simulink model "Modele_Projet_H2026_Gabarit"  (R2021a)
settings: Solver=FixedStepAuto  StartTime=0.0  StopTime=60  FixedStep=10e-6  RelTol=1e-3
InitFcn:
  | clear all
  | close all
  | 
  | % Chariot
  | 
  | M = 2.5 % [kg]
  | 
  | % Reducteur  / roue
  | 
  | G1 = 20        %  Rapport rédcuteur
  | r1  = 0.125     %  Rayon roue [m]
  | 
  | %Moteur 80ZYTC102-1 Brush DC Motor
  | 
  | uB = 24 % V
  | 
  | km = 0.0742   % Nm/A
  | 
  | kv =  0.0742 % V / (rad/s)
  | 
  | Lm = 1.577e-3 % H
  | 
  | Rm = 1.3    % Ohm
  | 
  | Jr = 1.5580e-04    % kg-m2
  | 
  | Jch =  M*r1^2/G1^2
  | 
  | Jm = Jr + Jch
  | 
  | Bm = 0.0015 % Nm.s
  | 
  | 
  | 
  | Cf = 300e-6  % F
  | 
  | Lf = 50e-6 %  H
  | 
  | Rf = 100000 % Ohm
  | 
  | 
  | % Couplage
  | k = 50   % Constante d'élasticité  [N/m]
  | 
  | 
  | 
  | % Parametre perso ajouté pour le test
  | 
  | 
  | uB = 24;            % [V]       Tension nominale de la batterie
  | 
  | 
  | %% -------------------------------------------------------------------------
  | %  2. MOTEUR À COURANT CONTINU  (80ZYTC102-1 Brush DC Motor)
  | %     Identique pour les deux chariots
  | %% -------------------------------------------------------------------------
  | Lm = 1.577e-3;      % [H]       Inductance de l'induit
  | Rm = 1.3;           % [Ohm]     Résistance de l'induit
  | km = 0.0742;        % [Nm/A]    Constante de couple
  | kv = 0.0742;        % [V.s/rad] Constante de tension (FEM)
  | Jr = 1.558e-4;      % [kg.m²]   Inertie du rotor (avec charge)
  | Bm = 1.5e-3;        % [Nm.s]    Coefficient de friction visqueuse
  | 
  | 
  | %% -------------------------------------------------------------------------
  | %  3. CHARIOT
  | %% -------------------------------------------------------------------------
  | M  = 2.5;           % [kg]      Masse d'un chariot
  | G  = 20;            % [-]       Rapport du réducteur de vitesse
  | r  = 0.125;         % [m]       Rayon des roues
  | 
  | 
  | %% -------------------------------------------------------------------------
  | %  4. FILTRE DU CONVERTISSEUR DE PUISSANCE
  | %% -------------------------------------------------------------------------
  | Cf = 300e-6;        % [F]       Condensateur du filtre
  | Lf = 50e-6;         % [H]       Inductance du filtre
  | Rf = 100e3;         % [Ohm]     Résistance du filtre
  | 
  | 
  | %% -------------------------------------------------------------------------
  | %  5. BANDE ÉLASTIQUE
  | %% -------------------------------------------------------------------------
  | k_elas = 50;        % [N/m]     Constante d'élasticité de la bande
  | L_band = 1;         % [m]       Longueur de la bande élastique
  | 
  | 
  | %% -------------------------------------------------------------------------
  | %  6. PARAMÈTRES CALCULÉS
  | %% -------------------------------------------------------------------------
  | 
  | 
  | % --- Inertie équivalente vue par le moteur (Éq. 4) ---
  | rG   = r / G;                           % [m/rad]   Gain cinématique = 0.00625
  | Jm   = Jr + M * rG^2;                   % [kg.m²]   = 2.535e-4
  | 
  | 
  | % --- Constantes de temps du moteur ---
  | tau_e = Lm / Rm;                        % [s]       Cste de temps électrique = 1.213e-3 s
  | tau_m = Jm / Bm;                        % [s]       Cste de temps mécanique  = 0.1690  s
  | 
  | 
  | % --- Produit des constantes moteur (FEM contre-réaction) ---
  | km_kv = km * kv;                        % [V.Nm/A²] = 5.506e-3
  | 
  | 
  | % --- Paramètres du modèle simplifié (tau_e négligé) ---
  | Bm_star  = Bm + km*kv/Rm;              % [Nm.s]    Friction équivalente = 5.737e-3
  | tau_m_st = Jm / Bm_star;               % [s]       Cste de temps simplifiée = 0.04418 s
  | Kv       = uB*km / (Rm * Bm_star);     % [rad/s]   Gain BO vitesse simplifié = 238.8
  | Kp       = Kv * rG;                     % [m/s]     Gain BO position simplifiée = 1.493
  | 
  | 
  | % --- Gain du convertisseur (simplifié) ---
  | K_conv = uB;                            % [V]       = 24  (gain pur)
  | 
  | 
  | % --- Gain cinématique couplage ---
  | rG_sq  = rG^2;
undefined symbols (not defined in the file or in its folder): sigbuilder_block
settings Model: Creator=cardenas  LastModifiedBy=arman

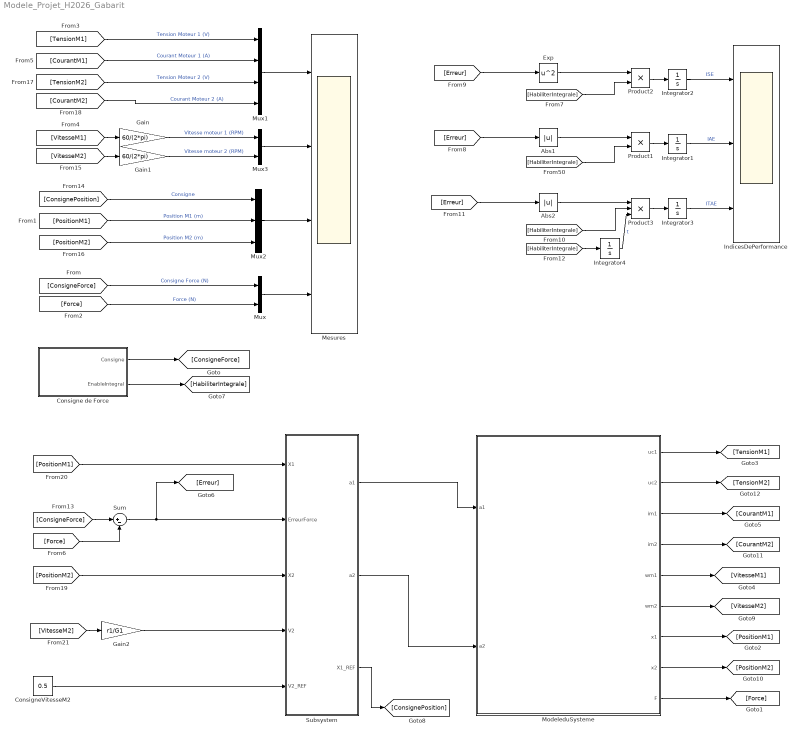
== system Modele_Projet_H2026_Gabarit ==
  Abs1 : Abs
  Abs2 : Abs
  Consigne de Force : Subsystem
  ConsigneVitesseM2 : Constant  Value=0.5
  Exp : Math  Operator=square  SaturateOnIntegerOverflow=on
  Gain : Gain  Gain=60/(2*pi)
  Gain1 : Gain  Gain=60/(2*pi)
  Gain2 : Gain  Gain=r1/G1
  IndicesDePerformance : Scope  NumInputPorts=3
  Integrator{1..4} (4 alike) : Integrator
  Mesures : Scope  NumInputPorts=4
  ModeleduSysteme : Subsystem
  Mux : Mux  Inputs=2
  Mux1 : Mux
  Mux2 : Mux  Inputs=3
  Mux3 : Mux  Inputs=2
  Product1 : Product
  Product2 : Product
  Product3 : Product  Inputs=3
  Subsystem : Subsystem
  Sum : Sum  Inputs=|+-
  wires:
  Mux/1 -> Mesures/4
  [ConsigneForce] -> Mux/1  "Consigne Force (N)"
  [PositionM1] -> Mux2/2  "Position M1 (m)"
  [Force] -> Mux/2  "Force (N)"
  [TensionM1] -> Mux1/1  "Tension Moteur 1 (V)"
  [VitesseM1] -> Gain/1
  Sum/1 -> [Erreur], Subsystem/2(ErreurForce)
  ModeleduSysteme/9(F) -> [Force]
  ModeleduSysteme/1(uc1) -> [TensionM1]
  ModeleduSysteme/7(x1) -> [PositionM1]
  ModeleduSysteme/3(im1) -> [CourantM1]
  [CourantM1] -> Mux1/2  "Courant Moteur 1 (A)"
  Mux1/1 -> Mesures/1
  ModeleduSysteme/5(wm1) -> [VitesseM1]
  [Force] -> Sum/2
  Gain/1 -> Mux3/1  "Vitesse moteur 1 (RPM)"
  [Erreur] -> Abs1/1
  [HabiliterIntegrale] -> Product1/2
  Abs1/1 -> Product1/1
  Product1/1 -> Integrator1/1
  Integrator1/1 -> IndicesDePerformance/2  "IAE"
  Product2/1 -> Integrator2/1
  Exp/1 -> Product2/1
  [HabiliterIntegrale] -> Product2/2
  Integrator2/1 -> IndicesDePerformance/1  "ISE"
  [Erreur] -> Exp/1
  Integrator3/1 -> IndicesDePerformance/3  "ITAE"
  Product3/1 -> Integrator3/1
  Abs2/1 -> Product3/1
  [HabiliterIntegrale] -> Product3/2
  [Erreur] -> Abs2/1
  Consigne de Force/2(EnableIntegral) -> [HabiliterIntegrale]
  [HabiliterIntegrale] -> Integrator4/1
  Integrator4/1 -> Product3/3  "t"
  [ConsigneForce] -> Sum/1
  [ConsignePosition] -> Mux2/1  "Consigne"
  Mux2/1 -> Mesures/3
  ModeleduSysteme/6(wm2) -> [VitesseM2]
  Mux3/1 -> Mesures/2
  Gain1/1 -> Mux3/2  "Vitesse moteur 2 (RPM)"
  [VitesseM2] -> Gain1/1
  ModeleduSysteme/8(x2) -> [PositionM2]
  [PositionM2] -> Mux2/3  "Position M2 (m)"
  ModeleduSysteme/4(im2) -> [CourantM2]
  ModeleduSysteme/2(uc2) -> [TensionM2]
  [TensionM2] -> Mux1/3  "Tension Moteur 2 (V)"
  [CourantM2] -> Mux1/4  "Courant Moteur 2 (A)"
  Consigne de Force/1(Consigne) -> [ConsigneForce]
  [VitesseM2] -> Gain2/1
  [PositionM1] -> Subsystem/1(X1)
  [PositionM2] -> Subsystem/3(X2)
  Gain2/1 -> Subsystem/4(V2)
  ConsigneVitesseM2/1 -> Subsystem/5(V2_REF)
  Subsystem/1(a1) -> ModeleduSysteme/1(a1)
  Subsystem/2(a2) -> ModeleduSysteme/2(a2)
  Subsystem/3(X1_REF) -> [ConsignePosition]

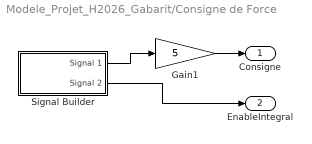
== system Modele_Projet_H2026_Gabarit/Consigne de Force ==
  Gain1 : Gain  Gain=5
  Signal Builder : Subsystem  Tag=STV Subsys  LoadFcn=sigbuilder_block('load');  StartFcn=sigbuilder_block('start');  StopFcn=sigbuilder_block('stop');  ClipboardFcn=sigbuilder_block('clipboard');  mask(Sigbuilder block){tuvar=[0:10]}
      mask help: Simulink:masks:SigbuilderBlock_MD
      mask init:
      | if ~strcmp(get_param(bdroot(gcbh),'SimulationStatus'),'stopped') tuvar = sigbuilder_block('maskInit'); end
      settings: CopyFcn=sigbuilder_block('copy');  DeleteFcn=sigbuilder_block('delete');  ModelCloseFcn=sigbuilder_block('modelClose');  PreSaveFcn=sigbuilder_block('preSave');  PauseFcn=sigbuilder_block('pause');  ContinueFcn=sigbuilder_block('continue');  NameChangeFcn=sigbuilder_block('namechange');  OpenFcn=sigbuilder_block('open',[138 164.25 838.5 442.5 ]);  CloseFcn=sigbuilder_block('close');
      mask Display: plot(0, 0, 100, 100,[2, 2, 32, 32, 2], [68, 8, 8, 68, 68],[32, 2], [38, 38], [32, 19, 2],[53, 60, 44], [32, 17, 17, 2],[16, 16, 31, 31]);txt = getActiveGroup(gcbh);text(2, 100, txt,'verticalAlignment', 'top');
  Consigne : Outport
  EnableIntegral : Outport  Port=2
  wires:
  Signal Builder/1(Signal 1) -> Gain1/1
  Gain1/1 -> Consigne/1
  Signal Builder/2(Signal 2) -> EnableIntegral/1

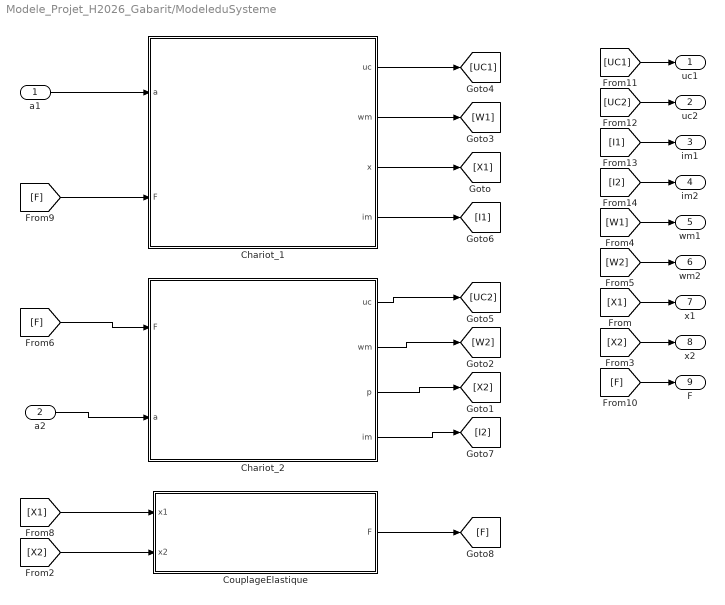
== system Modele_Projet_H2026_Gabarit/ModeleduSysteme ==
  a1 : Inport
  a2 : Inport  Port=2
  Chariot_1 : Subsystem
  Chariot_2 : Subsystem
  CouplageElastique : Subsystem
  uc1 : Outport
  uc2 : Outport  Port=2
  im1 : Outport  Port=3
  im2 : Outport  Port=4
  wm1 : Outport  Port=5
  wm2 : Outport  Port=6
  x1 : Outport  Port=7
  x2 : Outport  Port=8
  F : Outport  Port=9
  wires:
  CouplageElastique/1(F) -> [F]
  [X1] -> x1/1
  [X2] -> CouplageElastique/2(x2)
  [X2] -> x2/1
  [W1] -> wm1/1
  [W2] -> wm2/1
  Chariot_2/1(uc) -> [UC2]
  Chariot_2/2(wm) -> [W2]
  Chariot_2/3(p) -> [X2]
  Chariot_2/4(im) -> [I2]
  [F] -> Chariot_2/1(F)
  a2/1 -> Chariot_2/2(a)
  [X1] -> CouplageElastique/1(x1)
  [F] -> Chariot_1/2(F)
  Chariot_1/1(uc) -> [UC1]
  Chariot_1/2(wm) -> [W1]
  Chariot_1/3(x) -> [X1]
  Chariot_1/4(im) -> [I1]
  a1/1 -> Chariot_1/1(a)
  [F] -> F/1
  [UC1] -> uc1/1
  [UC2] -> uc2/1
  [I1] -> im1/1
  [I2] -> im2/1

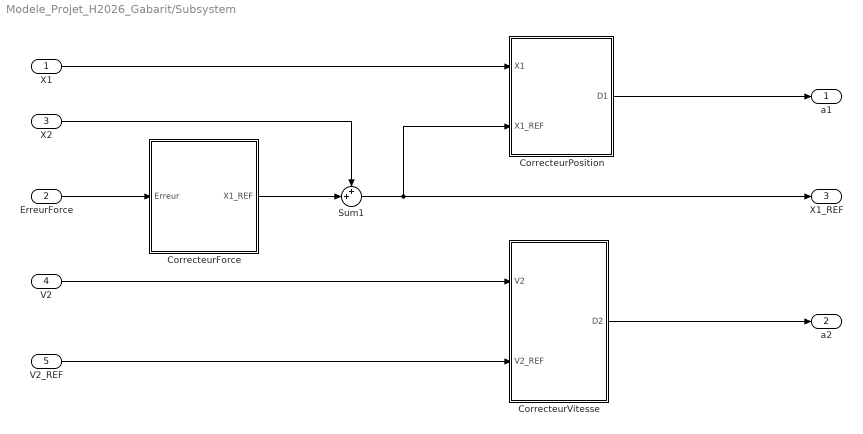
== system Modele_Projet_H2026_Gabarit/Subsystem ==
  X1 : Inport
  ErreurForce : Inport  Port=2
  X2 : Inport  Port=3
  V2 : Inport  Port=4
  V2_REF : Inport  Port=5
  CorrecteurForce : Subsystem
  CorrecteurPosition : Subsystem
  CorrecteurVitesse : Subsystem
  Sum1 : Sum  Inputs=++|
  a1 : Outport
  a2 : Outport  Port=2
  X1_REF : Outport  Port=3
  wires:
  CorrecteurPosition/1(D1) -> a1/1
  Sum1/1 -> X1_REF/1, CorrecteurPosition/2(X1_REF)
  CorrecteurVitesse/1(D2) -> a2/1
  CorrecteurForce/1(X1_REF) -> Sum1/2
  ErreurForce/1 -> CorrecteurForce/1(Erreur)
  X1/1 -> CorrecteurPosition/1(X1)
  V2/1 -> CorrecteurVitesse/1(V2)
  V2_REF/1 -> CorrecteurVitesse/2(V2_REF)
  X2/1 -> Sum1/1

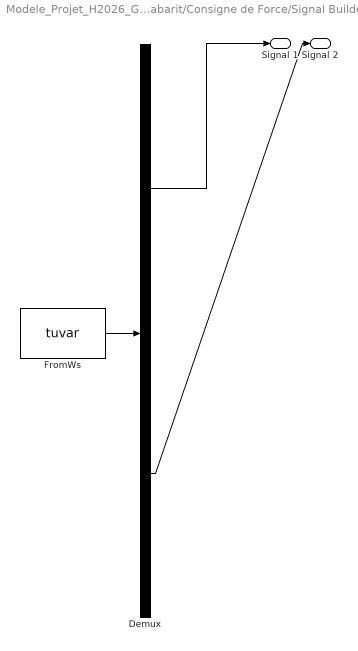
== system Modele_Projet_H2026_Gabarit/Consigne de Force/Signal Builder ==
  Demux : Demux  Tag=STV Demux  Outputs=2
      settings: DisplayOption=none
  FromWs : FromWorkspace  Tag=STV FromWs  VariableName=tuvar
      SigBuilderData=|
      | common.afterFinalStr = 'Extrapolate'
      | common.sampleTime = 0
      | dataSet.timeRange = [0 200]
      | dataSet.name = 'Group 1'
      | sbobj.Groups.Name = 'Group 1'
      | sbobj.Groups.Signals(1).Name = 'Signal 1'
      | sbobj.Groups.Signals(1).XData = [0 10 30 30 200]
      | sbobj.Groups.Signals(1).YData = [0 1 1 1.1 1.1]
      | sbobj.Groups.Signals(2).Name = 'Signal 2'
      | sbobj.Groups.Signals(2).XData = [0 30 30 200]
      | sbobj.Groups.Signals(2).YData = [0 0 1 1]
      | sbobj.Groups.TimeRange = [0 200]
  Signal 1 : Outport  Tag=STV Outport
  Signal 2 : Outport  Tag=STV Outport  Port=2
  wires:
  Demux/1 -> Signal 1/1
  FromWs/1 -> Demux/1
  Demux/2 -> Signal 2/1

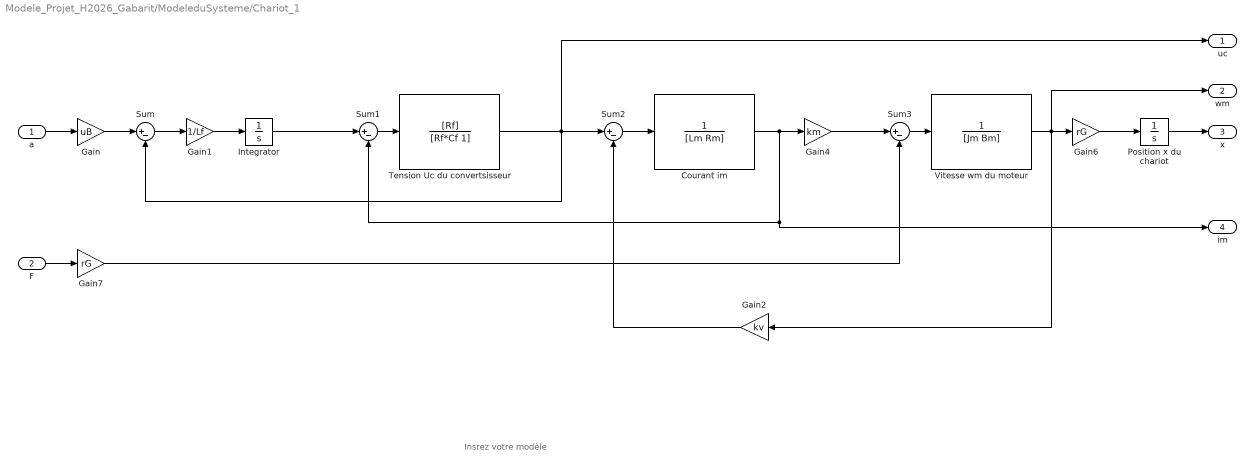
== system Modele_Projet_H2026_Gabarit/ModeleduSysteme/Chariot_1 ==
  note: Insrez votre modèle
  a : Inport
  F : Inport  Port=2
  "Courant im " : TransferFcn  Denominator=[Lm Rm]
  Gain : Gain  Gain=uB
  Gain1 : Gain  Gain=1/Lf
  Gain2 : Gain  Gain=kv
  Gain4 : Gain  Gain=km
  Gain6 : Gain  Gain=rG
  Gain7 : Gain  Gain=rG
  Integrator : Integrator
  Position x du chariot : Integrator
  Sum{,1..3} (4 alike) : Sum  Inputs=|+-
  Tension Uc du convertsisseur : TransferFcn  Numerator=[Rf]  Denominator=[Rf*Cf 1]
  Vitesse wm du moteur : TransferFcn  Denominator=[Jm Bm]
  uc : Outport
  wm : Outport  Port=2
  x : Outport  Port=3
  im : Outport  Port=4
  wires:
  Gain/1 -> Sum/1
  Sum/1 -> Gain1/1
  Gain4/1 -> Sum3/1
  Gain1/1 -> Integrator/1
  Integrator/1 -> Sum1/1
  Sum1/1 -> Tension Uc du convertsisseur/1
  Tension Uc du convertsisseur/1 -> Sum/2, Sum2/1, uc/1
  Sum2/1 -> "Courant im "/1
  "Courant im "/1 -> im/1, Sum1/2, Gain4/1
  Sum3/1 -> Vitesse wm du moteur/1
  Vitesse wm du moteur/1 -> wm/1, Gain2/1, Gain6/1
  Gain6/1 -> Position x du chariot/1
  Position x du chariot/1 -> x/1
  Gain7/1 -> Sum3/2
  Gain2/1 -> Sum2/2
  a/1 -> Gain/1
  F/1 -> Gain7/1

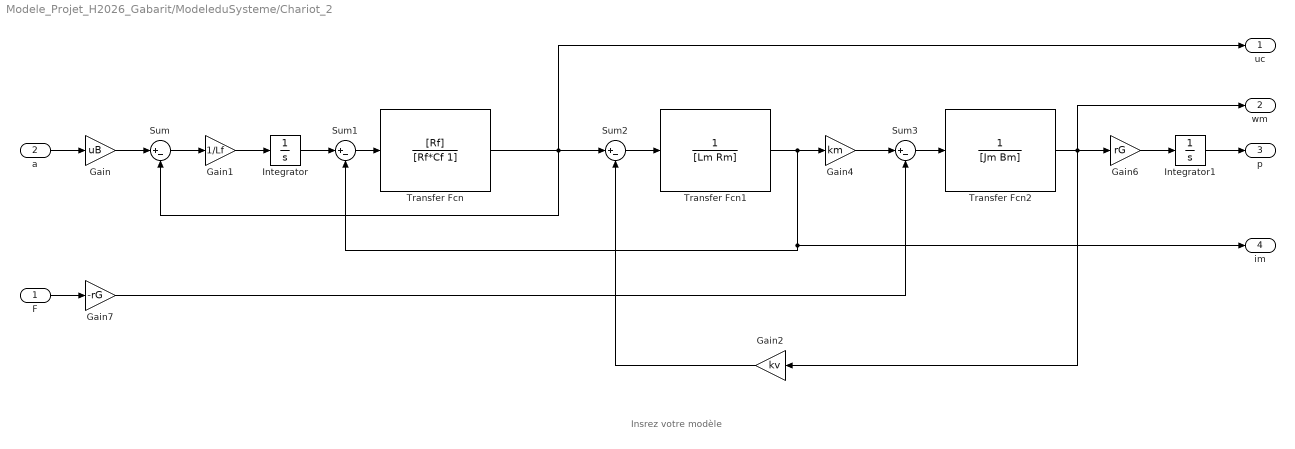
== system Modele_Projet_H2026_Gabarit/ModeleduSysteme/Chariot_2 ==
  note: Insrez votre modèle
  F : Inport
  a : Inport  Port=2
  Gain : Gain  Gain=uB
  Gain1 : Gain  Gain=1/Lf
  Gain2 : Gain  Gain=kv
  Gain4 : Gain  Gain=km
  Gain6 : Gain  Gain=rG
  Gain7 : Gain  Gain=-rG
  Integrator : Integrator
  Integrator1 : Integrator
  Sum{,1..3} (4 alike) : Sum  Inputs=|+-
  Transfer Fcn : TransferFcn  Numerator=[Rf]  Denominator=[Rf*Cf 1]
  Transfer Fcn1 : TransferFcn  Denominator=[Lm Rm]
  Transfer Fcn2 : TransferFcn  Denominator=[Jm Bm]
  uc : Outport
  wm : Outport  Port=2
  p : Outport  Port=3
  im : Outport  Port=4
  wires:
  Gain2/1 -> Sum2/2
  Sum3/1 -> Transfer Fcn2/1
  Transfer Fcn1/1 -> Sum1/2, im/1, Gain4/1
  Sum2/1 -> Transfer Fcn1/1
  Gain6/1 -> Integrator1/1
  Transfer Fcn2/1 -> Gain6/1, wm/1, Gain2/1
  Sum1/1 -> Transfer Fcn/1
  Transfer Fcn/1 -> uc/1, Sum/2, Sum2/1
  Gain1/1 -> Integrator/1
  Gain7/1 -> Sum3/2
  F/1 -> Gain7/1
  a/1 -> Gain/1
  Integrator1/1 -> p/1
  Sum/1 -> Gain1/1
  Integrator/1 -> Sum1/1
  Gain/1 -> Sum/1
  Gain4/1 -> Sum3/1

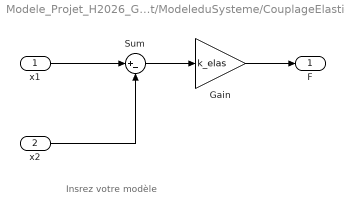
== system Modele_Projet_H2026_Gabarit/ModeleduSysteme/CouplageElastique ==
  note: Insrez votre modèle
  x1 : Inport
  x2 : Inport  Port=2
  Gain : Gain  Gain=k_elas
  Sum : Sum  Inputs=|+-
  F : Outport
  wires:
  x2/1 -> Sum/2
  x1/1 -> Sum/1
  Sum/1 -> Gain/1
  Gain/1 -> F/1

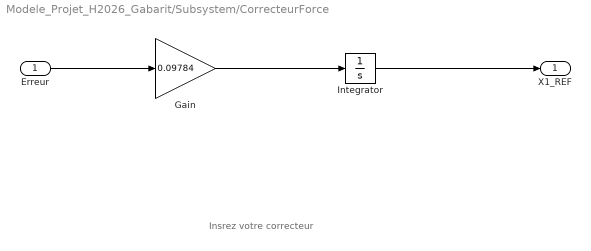
== system Modele_Projet_H2026_Gabarit/Subsystem/CorrecteurForce ==
  note: Insrez votre correcteur
  Erreur : Inport
  Gain : Gain  Gain=0.09784
  Integrator : Integrator
  X1_REF : Outport
  wires:
  Gain/1 -> Integrator/1
  Integrator/1 -> X1_REF/1
  Erreur/1 -> Gain/1

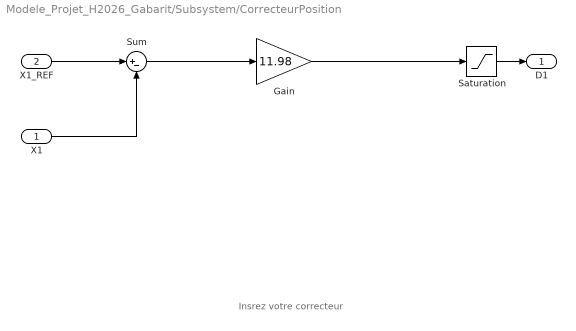
== system Modele_Projet_H2026_Gabarit/Subsystem/CorrecteurPosition ==
  note: Insrez votre correcteur
  X1 : Inport
  X1_REF : Inport  Port=2
  Gain : Gain  Gain=11.98
  Saturation : Saturate  UpperLimit=1  LowerLimit=-1
  Sum : Sum  Inputs=|+-
  D1 : Outport
  wires:
  X1/1 -> Sum/2
  Saturation/1 -> D1/1
  X1_REF/1 -> Sum/1
  Sum/1 -> Gain/1
  Gain/1 -> Saturation/1

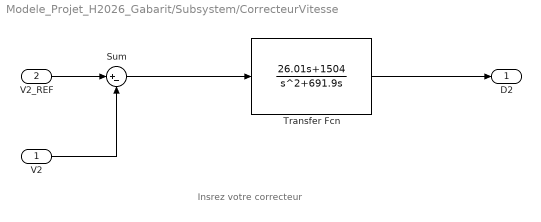
== system Modele_Projet_H2026_Gabarit/Subsystem/CorrecteurVitesse ==
  note: Insrez votre correcteur
  V2 : Inport
  V2_REF : Inport  Port=2
  Sum : Sum  Inputs=|+-
  Transfer Fcn : TransferFcn  Numerator=[26.01 1504]  Denominator="[1 691.9  0]"
  D2 : Outport
  wires:
  V2_REF/1 -> Sum/1
  V2/1 -> Sum/2
  Sum/1 -> Transfer Fcn/1
  Transfer Fcn/1 -> D2/1
